simulink model "qdrdac"  (R2012b)
settings: Solver=ode45  StartTime=0.0  StopTime=100  RelTol=1e-3
undefined symbols (not defined in the file or in its folder): pfb_coeff_gen_calc, sfp
undefined symbols (not defined in the file): SL, transtable
libraries: xbsIndex_r4 x4366, casper_library_misc x73, xps_library x14, casper_library_delays x12, maddogLibrary x4, simulink x2
(part 4 of 45)

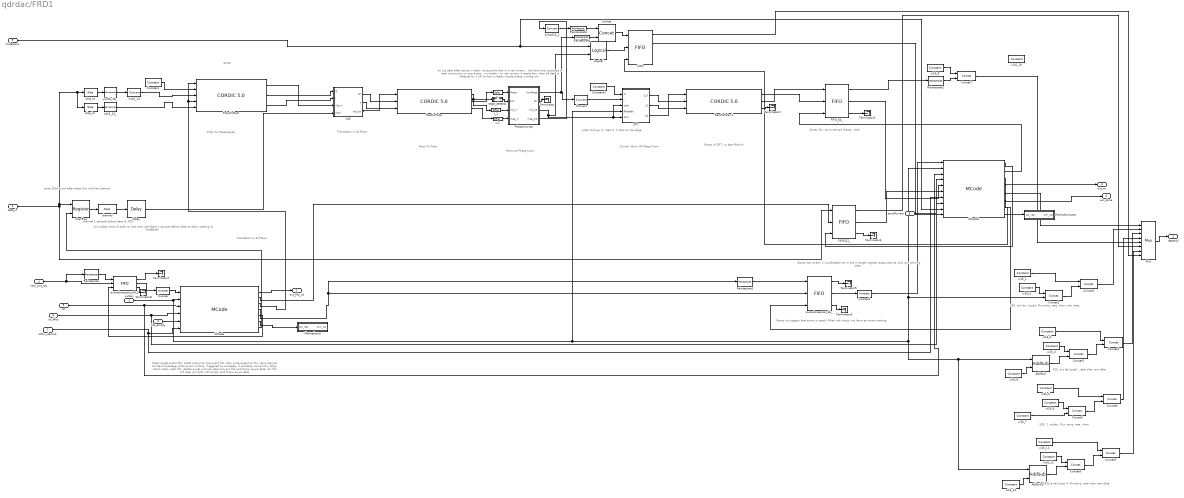
== system qdrdac/FRD1 ==
  note: stroe 32bit word after aaaa
      | this wird has channel
  note: 20 is delay time of polar to rect
      | chan get there 1 sample before data
      | to allow reading of theBRAM
  note: channel 1 sample before
      | data to FRD
  note: Z=20
  note: on 1st data after pause in data, we assume that is a new event...
      | the fsms are supposed to read continuous on one event...no breaks.
      | on new event, it resets fsm. then all data is delayed bu 1 clk so fsm
      | is ready insode phase unwrap ckt.
  note: 555, evt len type1 , aaa chan raw data
  note: 555, evt len, type3, fluxramp, aaa, chan, raw data
  note: 555, 2, evtlen, flux ramp, aaa, chan,
  note: Stores flux ramp dempd [hases. chan
  note: when dvld go hi, start it. it resp to rise edge
  note: Polar To Rectangular
  note: Translation in IQ Plane
  note: Remove Phase Jump
  note: Fourier Xform
      | Of Phase Term
  note: Rect To Polar
  note: Phase of DFT,
      | or Atan(Re/Im)
  note: Translation in IQ Plane
  note: Stores raw event.
      | 2 wordheader
      | len is the in length register
      | aaaa,chan,ts, and raw ph/mag data
  note: Stores up triggers that event is ready
      | When not mptuy we have en event waiting
  note: Read single event fifo.
      | Write output to 2nd event fifo.
      | Also write output to flux ramp demod ckt
      | Send message when event is done.
      | Triggered by evtready. if evtready come from fofop, clrevt ready read fifo.
      | delete evnet will just read sing evt fifo and throw awya data.
      | ckr fifo will clear evt fuifo intil empty and throw awya data
  note: 5555,evlen,type 4, fluxramp, aaa chan tran data
  evtlen : Inport
  fifo_empty : Inport  Port=2
  data_in : Inport  Port=3
  new_evt_rdy : Inport  Port=4
  rst : Inport  Port=5
  clr_fifos : Inport  Port=6
  isflux_demod : Inport  Port=7
  savefluxraw : Inport  Port=8
  circletrans : Inport  Port=9
  AddSub : xbsIndex_r4/AddSub  mode=Addition  use_carryin=off  use_carryout=off  en=off  latency=1  precision=User Defined  arith_type=Unsigned  n_bits=8  bin_pt=0  quantization=Truncate  overflow=Wrap  dbl_ovrd=off  use_behavioral_HDL=off  hw_selection=Fabric  pipelined=off  block_type=addsub
  AddSub1 : xbsIndex_r4/AddSub  mode=Addition  use_carryin=off  use_carryout=off  en=off  latency=1  precision=User Defined  arith_type=Unsigned  n_bits=8  bin_pt=0  quantization=Truncate  overflow=Wrap  dbl_ovrd=off  use_behavioral_HDL=off  hw_selection=Fabric  pipelined=off  block_type=addsub
  Concat{,1..9} (10 alike) : xbsIndex_r4/Concat  num_inputs=2  dbl_ovrd=off  block_type=concat
  Constant : xbsIndex_r4/Constant  const=0  gui_display_data_type=Fixed-point  arith_type=Signed (2's comp)  n_bits=16  bin_pt=14  preci_type=Single  exp_width=8  frac_width=24  explicit_period=on  period=1  equ=P=C  opselect=C  inp2=PCIN>>17  opr=+  inp1=P  carry=CIN  dbl_ovrd=off  block_type=constant
  Constant3 : xbsIndex_r4/Constant  const=0  gui_display_data_type=Fixed-point  arith_type=Signed (2's comp)  n_bits=16  bin_pt=14  preci_type=Single  exp_width=8  frac_width=24  explicit_period=on  period=1  equ=P=C  opselect=C  inp2=PCIN>>17  opr=+  inp1=P  carry=CIN  dbl_ovrd=off  block_type=constant
  Convert : xbsIndex_r4/Convert  gui_display_data_type=Fixed-point  arith_type="Signed  (2's comp)"  n_bits=16  bin_pt=14  float_type=Single  exp_bits=8  fraction_bits=24  quantization=Truncate  overflow=Wrap  en=off  latency=0  dbl_ovrd=off  pipeline=off  block_type=convert
  DFT : Subsystem
  Delay : xbsIndex_r4/Delay  rst=off  infoeditControl=Selection of Reset will increase slice count due to use of real FFs and instead of SRLs  en=off  latency=19  dbl_ovrd=off  reg_retiming=off  block_type=delay
  FIFO : xbsIndex_r4/FIFO  mem_type=Block RAM  performance_options=First_Word_Fall_Through  infoedit1=Available only for V4, V5, V6, V7, K7, A7 and Zynq devices.  embedded_registers=off  depth=512  percent_nbits=1  rst=off  en=off  use_dcount=off  use_percent_full_port=on  use_almost_empty=off  almost_empty_thresh=2  use_almost_full=off  almost_full_thresh=14  dbl_ovrd=off  explicit_period=off  block_type=fifo
  FIFO512_ : xbsIndex_r4/FIFO  mem_type=Block RAM  performance_options=First_Word_Fall_Through  infoedit1=Available only for V4, V5, V6, V7, K7, A7 and Zynq devices.  embedded_registers=off  depth=512  percent_nbits=1  rst=off  en=off  use_dcount=off  use_percent_full_port=off  use_almost_empty=off  almost_empty_thresh=2  use_almost_full=off  almost_full_thresh=256  dbl_ovrd=off  explicit_period=off  block_type=fifo
  FIFO_64_ : xbsIndex_r4/FIFO  mem_type=Block RAM  performance_options=First_Word_Fall_Through  infoedit1=Available only for V4, V5, V6, V7, K7, A7 and Zynq devices.  embedded_registers=off  depth=64  percent_nbits=1  rst=off  en=off  use_dcount=off  use_percent_full_port=off  use_almost_empty=off  almost_empty_thresh=2  use_almost_full=off  almost_full_thresh=32  dbl_ovrd=off  explicit_period=off  block_type=fifo
  Inverter : xbsIndex_r4/Inverter  en=off  latency=0  dbl_ovrd=off  block_type=inv
  Inverter1 : xbsIndex_r4/Inverter  en=off  latency=0  dbl_ovrd=off  block_type=inv
  Logical : xbsIndex_r4/Logical  logical_function=AND  inputs=2  en=off  latency=0  precision=Full  arith_type=Unsigned  n_bits=16  bin_pt=0  align_bp=on  dbl_ovrd=off  block_type=logical
  MCode : xbsIndex_r4/MCode  mfname=fluxRampFSM.m  explicit_period=off  period=1  inputsTable={'boundInpExpr'=>['','','','','',''],'inputs'=>['event_rdy','event_length','rst','clr_fifos','fifo_empty','is_fluxrampdemod']}  outputsTable={'outputs'=>['eventfifo_rd','outfifo_wr','demod_wr','event_done','clr_evt_rdy','stout'],'suppressOut'=>['off','off','off','off','off','off']}  dbl_ovrd=off  enable_stdout=off  enable_debug=off  suppress_output=on  defparams={}  hide_port_list={}  block_type=mcode
  MCode1 : xbsIndex_r4/MCode  mfname=fluxRampFSMOut2  explicit_period=on  period=1  inputsTable={'boundInpExpr'=>['','','','','','','',''],'inputs'=>['event_rdy','event_length','rst','clr_fifos','rawevt_fifo_empty','fluxrmp_fifo_empy','is_fluxrampdemod','is_savefluxraw']}  outputsTable={'outputs'=>['eventfifo_rd','fluxfifo_rd','outfifo_wr','wr_select','event_done','clr_evt_rdy','stout'],'suppressOut'=>['off','off','off','off','off','off','off']}  dbl_ovrd=off  enable_stdout=off  enable_debug=off  suppress_output=on  defparams={}  hide_port_list={}  block_type=mcode
  Mux : xbsIndex_r4/Mux  inputs=7  en=off  latency=0  precision=Full  arith_type=Unsigned  n_bits=16  bin_pt=14  quantization=Truncate  overflow=Wrap  dbl_ovrd=off  block_type=mux
  PhaseUnwrap : Subsystem
  "PolarToRect " : xbsIndex_r4/CORDIC 5.0   functional_selection=Rotate  architectural_configuration=Parallel  pipelining_mode=Maximum  data_format=SignedFraction  phase_format=Scaled_Radians  input_width=16  output_width=16  round_mode=Truncate  iterations=0  precision=0  compensation_scaling=Embedded_Multiplier  coarse_rotation=on  aclken=off  aresetn=off  out_tready=off  cartesian_has_tuser=off  cartesian_has_tlast=off  cartesian_tuser_width=1  phase_has_tuser=off  phase_has_tlast=off  phase_tuser_width=1  out_tlast_behv=Null  flow_control=NonBlocking  optimize_goal=Performance  trim_axipin_name=on  ip_name=CORDIC  ip_version=5.0  dsptool_ready=true  ipcore_usecache=true  ipcore_useipmodelcache=true  wrapper_available=true  port_translation_map={ 'aclken' => 'en', 'aresetn' => 'rst' }  block_type=cordic_v5_0
      settings: infoedit=CORDIC 5.0
  "RectToPolar " : xbsIndex_r4/CORDIC 5.0   functional_selection=Translate  architectural_configuration=Parallel  pipelining_mode=Maximum  data_format=SignedFraction  phase_format=Scaled_Radians  input_width=16  output_width=16  round_mode=Truncate  iterations=0  precision=0  compensation_scaling=Embedded_Multiplier  coarse_rotation=on  aclken=off  aresetn=off  out_tready=off  cartesian_has_tuser=off  cartesian_has_tlast=off  cartesian_tuser_width=1  phase_has_tuser=off  phase_has_tlast=off  phase_tuser_width=1  out_tlast_behv=Null  flow_control=NonBlocking  optimize_goal=Performance  trim_axipin_name=on  ip_name=CORDIC  ip_version=5.0  dsptool_ready=true  ipcore_usecache=true  ipcore_useipmodelcache=true  wrapper_available=true  port_translation_map={ 'aclken' => 'en', 'aresetn' => 'rst' }  block_type=cordic_v5_0
      settings: infoedit=CORDIC 5.0
  RectToPolar 1 : xbsIndex_r4/CORDIC 5.0   functional_selection=Translate  architectural_configuration=Parallel  pipelining_mode=Maximum  data_format=SignedFraction  phase_format=Scaled_Radians  input_width=16  output_width=16  round_mode=Truncate  iterations=0  precision=0  compensation_scaling=Embedded_Multiplier  coarse_rotation=on  aclken=off  aresetn=off  out_tready=off  cartesian_has_tuser=off  cartesian_has_tlast=off  cartesian_tuser_width=1  phase_has_tuser=off  phase_has_tlast=off  phase_tuser_width=1  out_tlast_behv=Null  flow_control=NonBlocking  optimize_goal=Performance  trim_axipin_name=on  ip_name=CORDIC  ip_version=5.0  dsptool_ready=true  ipcore_usecache=true  ipcore_useipmodelcache=true  wrapper_available=true  port_translation_map={ 'aclken' => 'en', 'aresetn' => 'rst' }  block_type=cordic_v5_0
      settings: infoedit=CORDIC 5.0
  Reinterpret : xbsIndex_r4/Reinterpret  force_arith_type=on  arith_type=Unsigned  force_bin_pt=off  bin_pt=0  block_type=reinterpret
  Reinterpret1 : xbsIndex_r4/Reinterpret  force_arith_type=on  arith_type=Unsigned  force_bin_pt=off  bin_pt=0  block_type=reinterpret
  Reinterpret2 : xbsIndex_r4/Reinterpret  force_arith_type=on  arith_type=Unsigned  force_bin_pt=on  bin_pt=0  block_type=reinterpret
  Reinterpret3 : xbsIndex_r4/Reinterpret  force_arith_type=on  arith_type=Unsigned  force_bin_pt=on  bin_pt=0  block_type=reinterpret
  Reinterpret4 : xbsIndex_r4/Reinterpret  force_arith_type=on  arith_type=Unsigned  force_bin_pt=on  bin_pt=0  block_type=reinterpret
  Terminator{,2..8} (8 alike) : Terminator
  chanReg : xbsIndex_r4/Register  init=0  rst=off  en=on  dbl_ovrd=off  block_type=register
  channel : xbsIndex_r4/Slice  nbits=8  boolean_output=off  mode=Lower Bit Location + Width  bit1=0  base1=MSB of Input  bit0=0  base0=LSB of Input  dbl_ovrd=off  block_type=slice
  edge_detect1 : Subsystem  AncestorBlock=casper_library_misc/edge_detect  mask(edge_detect){edge=Rising, polarity=Active High, x_in=[0 0.08 0.08 0.16 0.16 0.24 0.24 0.32 0.32 0.4], y_in=[-1 -1  1  1  1  1  1  1  1  1], x_out=[0.6 0.68 0.68 0.76 0.76 0.84 0.84 0.92 0.92 1], y_out=[-1 -1  1  1 -1 -1 -1 -1 -1 -1]}
      mask prompts: edge "Edge Type"; polarity "Output Polarity"; x_in "Input X Positions"; y_in "Input Y Positions"; x_out "Output X Positions"; y_out "Output Y Positions"
      mask help: Output is active for one-cycle after each edge of the specified type (i.e. rising, falling or both).
      mask init: same as qdrdac/FRD/edge_detect1
      settings: AttributesFormatString=|
      | rising edges
      | active high
      mask Help: Output is active for one-cycle after each edge of the specified type (i.e. rising, falling, or both).  Latency is zero.
      mask TypeOptions edge: Rising | Falling | Both
      mask TypeOptions polarity: Active High | Active Low
      mask Display:
      | plot(x_in_num,0.5+y_in_num*0.2);
      | plot(x_out_num,0.5+y_out_num*0.2);
  evendonequtut_64_ : xbsIndex_r4/FIFO  mem_type=Block RAM  performance_options=First_Word_Fall_Through  infoedit1=Available only for V4, V5, V6, V7, K7, A7 and Zynq devices.  embedded_registers=off  depth=16  percent_nbits=1  rst=off  en=off  use_dcount=off  use_percent_full_port=off  use_almost_empty=off  almost_empty_thresh=2  use_almost_full=off  almost_full_thresh=14  dbl_ovrd=off  explicit_period=off  block_type=fifo
  evendonequtut_64_1 : xbsIndex_r4/FIFO  mem_type=Block RAM  performance_options=First_Word_Fall_Through  infoedit1=Available only for V4, V5, V6, V7, K7, A7 and Zynq devices.  embedded_registers=off  depth=16  percent_nbits=1  rst=off  en=off  use_dcount=off  use_percent_full_port=off  use_almost_empty=off  almost_empty_thresh=2  use_almost_full=off  almost_full_thresh=14  dbl_ovrd=off  explicit_period=off  block_type=fifo
  flrampfsmoutst : Subsystem  Tag=xps:sw_reg  AncestorBlock=xps_library/software register  mask(swreg){mode=one value, io_dir=To Processor, io_delay=0, sample_period=1, names=reg, bitwidths=5, arith_types=0, bin_pts=0, sim_port=on, show_format=off}
      mask prompts: io_dir "I/O direction"; io_delay "I/O delay"; sample_period "Sample period"; names "Name:"; bitwidths "Bitwidth:"; arith_types "Type (ufix=0, fix=1, bool=2):"; bin_pts "Binary pt:"; sim_port "Provide sim input/output?"; show_format "Print format string?"
      mask init:
      | swreg_init(gcb)
      settings: AttributesFormatString=1output
      mask TypeOptions mode: one value | fields of equal size | fields of arbitrary size
      mask Callback mode: swreg_cb(gcb);
      mask TypeOptions io_dir: To Processor | From Processor
      mask Callback io_dir:
      | mask_enables = get_param(gcb, 'MaskEnables');
      | mask_names = get_param(gcb, 'MaskNames');
      | if strcmp(get_param(gcb, 'io_dir'), 'To Processor'),
      |     mask_enables{ismember(mask_names, 'sample_period')} = 'off';
      | else
      |     mask_enables{ismember(mask_names, 'sample_period')} = 'on';
      | end
      | set_param(gcb, 'MaskEnables', mask_enables);
      mask Callback bitwidths:
      | swreg_maskcheck(gcb);
      | % blk = gcb;
      | % mode = get_param(blk, 'mode');
      | % current_widths = eval(get_param(blk, 'bitwidths'));
      | % if (strcmp(mode, 'one value') || strcmp(mode, 'fields of equal size')) && (length(current_widths) > 1),
      | %     error('Only one width may be specified for this mode.');
      | % elseif strcmp(mode, 'fields of arbitrary size')
      | %     current_names = textscan(strtrim(strrep(strrep(get_param(blk, 'names'), ']', ''), '[', '')), '%s');
      | %     current_names = current_names{1};
      | %     numios = length(current_names);
      | %     if length(current_widths) ~= numios,
      | %         error('%d field names specified, but %d widths?', numios, length(current_widths));
      | %     end
      | % end
      | % total_width = 0;
      | % for ctr = 1 : length(current_widths),
      | %     total_width = total_width + current_widths(ctr);
      | % end
      | % if total_width > 32,
      | %     error('Total width must be 32 or less, set to %d.', total_width);
      | % end
      mask Callback arith_types:
      | [numios, ~, ~, ~, current_types] = swreg_maskcheck(gcb);
      | % blk = gcb;
      | % mode = get_param(blk, 'mode');
      | % current_types = eval(get_param(blk, 'arith_types'));
      | % numios = length(current_types);
      | % if (strcmp(mode, 'one value') || strcmp(mode, 'fields of equal size')) && (length(current_types) > 1),
      | %     error('Only one type may be specified for this mode.');
      | % elseif strcmp(mode, 'fields of arbitrary size')
      | %     current_names = textscan(strtrim(strrep(strrep(get_param(blk, 'names'), ']', ''), '[', '')), '%s');
      | %     current_names = current_names{1};
      | %     numios = length(current_names);
      | %     if length(current_types) ~= numios,
      | %         error('%d field names specified, but %d types?', numios, length(current_types));
      | %     end
      | % end
      | problem = 0;
      | for ctr = 1 : numios,
      |     t = current_types(ctr);
      |     if (t < 0) || (t > 2),
      |         problem = t;
      |         ctr = numios + 1;
      |     end
      | end
      | if problem ~= 0,
      |     error('Type cannot be %i, must be 0, 1 or 2.', problem);
      | end
      mask Callback bin_pts:
      | swreg_maskcheck(gcb);
      | % blk = gcb;
      | % mode = get_param(blk, 'mode');
      | % current_bins = eval(get_param(blk, 'bin_pts'));
      | % if (strcmp(mode, 'one value') || strcmp(mode, 'fields of equal size')) && (length(current_bins) > 1),
      | %     error('Only one binary pt may be specified for this mode.');
      | % elseif strcmp(mode, 'fields of arbitrary size')
      | %     current_names = textscan(strtrim(strrep(strrep(get_param(blk, 'names'), ']', ''), '[', '')), '%s');
      | %     current_names = current_names{1};
      | %     numios = length(current_names);
      | %     if length(current_bins) ~= numios,
      | %         error('%d field names specified, but %d binary pts?', numios, length(current_bins));
      | %     end
      | % end
  flrampfsmst : Subsystem  Tag=xps:sw_reg  AncestorBlock=xps_library/software register  mask(swreg){mode=one value, io_dir=To Processor, io_delay=0, sample_period=1, names=reg, bitwidths=4, arith_types=0, bin_pts=0, sim_port=on, show_format=off}
      mask prompts: io_dir "I/O direction"; io_delay "I/O delay"; sample_period "Sample period"; names "Name:"; bitwidths "Bitwidth:"; arith_types "Type (ufix=0, fix=1, bool=2):"; bin_pts "Binary pt:"; sim_port "Provide sim input/output?"; show_format "Print format string?"
      mask init:
      | swreg_init(gcb)
      settings: AttributesFormatString=1output
      mask TypeOptions mode: one value | fields of equal size | fields of arbitrary size
      mask Callback mode: swreg_cb(gcb);
      mask TypeOptions io_dir: To Processor | From Processor
      mask Callback io_dir:
      | mask_enables = get_param(gcb, 'MaskEnables');
      | mask_names = get_param(gcb, 'MaskNames');
      | if strcmp(get_param(gcb, 'io_dir'), 'To Processor'),
      |     mask_enables{ismember(mask_names, 'sample_period')} = 'off';
      | else
      |     mask_enables{ismember(mask_names, 'sample_period')} = 'on';
      | end
      | set_param(gcb, 'MaskEnables', mask_enables);
      mask Callback bitwidths:
      | swreg_maskcheck(gcb);
      | % blk = gcb;
      | % mode = get_param(blk, 'mode');
      | % current_widths = eval(get_param(blk, 'bitwidths'));
      | % if (strcmp(mode, 'one value') || strcmp(mode, 'fields of equal size')) && (length(current_widths) > 1),
      | %     error('Only one width may be specified for this mode.');
      | % elseif strcmp(mode, 'fields of arbitrary size')
      | %     current_names = textscan(strtrim(strrep(strrep(get_param(blk, 'names'), ']', ''), '[', '')), '%s');
      | %     current_names = current_names{1};
      | %     numios = length(current_names);
      | %     if length(current_widths) ~= numios,
      | %         error('%d field names specified, but %d widths?', numios, length(current_widths));
      | %     end
      | % end
      | % total_width = 0;
      | % for ctr = 1 : length(current_widths),
      | %     total_width = total_width + current_widths(ctr);
      | % end
      | % if total_width > 32,
      | %     error('Total width must be 32 or less, set to %d.', total_width);
      | % end
      mask Callback arith_types:
      | [numios, ~, ~, ~, current_types] = swreg_maskcheck(gcb);
      | % blk = gcb;
      | % mode = get_param(blk, 'mode');
      | % current_types = eval(get_param(blk, 'arith_types'));
      | % numios = length(current_types);
      | % if (strcmp(mode, 'one value') || strcmp(mode, 'fields of equal size')) && (length(current_types) > 1),
      | %     error('Only one type may be specified for this mode.');
      | % elseif strcmp(mode, 'fields of arbitrary size')
      | %     current_names = textscan(strtrim(strrep(strrep(get_param(blk, 'names'), ']', ''), '[', '')), '%s');
      | %     current_names = current_names{1};
      | %     numios = length(current_names);
      | %     if length(current_types) ~= numios,
      | %         error('%d field names specified, but %d types?', numios, length(current_types));
      | %     end
      | % end
      | problem = 0;
      | for ctr = 1 : numios,
      |     t = current_types(ctr);
      |     if (t < 0) || (t > 2),
      |         problem = t;
      |         ctr = numios + 1;
      |     end
      | end
      | if problem ~= 0,
      |     error('Type cannot be %i, must be 0, 1 or 2.', problem);
      | end
      mask Callback bin_pts:
      | swreg_maskcheck(gcb);
      | % blk = gcb;
      | % mode = get_param(blk, 'mode');
      | % current_bins = eval(get_param(blk, 'bin_pts'));
      | % if (strcmp(mode, 'one value') || strcmp(mode, 'fields of equal size')) && (length(current_bins) > 1),
      | %     error('Only one binary pt may be specified for this mode.');
      | % elseif strcmp(mode, 'fields of arbitrary size')
      | %     current_names = textscan(strtrim(strrep(strrep(get_param(blk, 'names'), ']', ''), '[', '')), '%s');
      | %     current_names = current_names{1};
      | %     numios = length(current_names);
      | %     if length(current_bins) ~= numios,
      | %         error('%d field names specified, but %d binary pts?', numios, length(current_bins));
      | %     end
      | % end
  int16_13_ : xbsIndex_r4/Reinterpret  force_arith_type=on  arith_type="Signed  (2's comp)"  force_bin_pt=on  bin_pt=13  block_type=reinterpret
      settings: block_version=9.1.01
  int16_14 : xbsIndex_r4/Convert  gui_display_data_type=Fixed-point  arith_type="Signed  (2's comp)"  n_bits=16  bin_pt=14  float_type=Single  exp_bits=8  fraction_bits=24  quantization=Truncate  overflow=Wrap  en=off  latency=0  dbl_ovrd=off  pipeline=off  block_type=convert
  slice_im : xbsIndex_r4/Slice  nbits=16  boolean_output=off  mode=Lower Bit Location + Width  bit1=0  base1=MSB of Input  bit0=0  base0=LSB of Input  dbl_ovrd=off  block_type=slice
      settings: block_version=9.1.01
  slice_re : xbsIndex_r4/Slice  nbits=16  boolean_output=off  mode=Upper Bit Location + Width  bit1=0  base1=MSB of Input  bit0=0  base0=LSB of Input  dbl_ovrd=off  block_type=slice
      settings: block_version=9.1.01
  trIQ : Subsystem
  ui16_{1..2,5,10..11} (5 alike) : xbsIndex_r4/Constant  const=21845  gui_display_data_type=Fixed-point  arith_type=Unsigned  n_bits=16  bin_pt=0  preci_type=Single  exp_width=8  frac_width=24  explicit_period=on  period=1  equ=P=C  opselect=C  inp2=PCIN>>17  opr=+  inp1=P  carry=CIN  dbl_ovrd=off  block_type=constant
  ui16_12 : xbsIndex_r4/Constant  const=4  gui_display_data_type=Fixed-point  arith_type=Unsigned  n_bits=8  bin_pt=0  preci_type=Single  exp_width=8  frac_width=24  explicit_period=on  period=1  equ=P=C  opselect=C  inp2=PCIN>>17  opr=+  inp1=P  carry=CIN  dbl_ovrd=off  block_type=constant
  ui16_13 : xbsIndex_r4/Constant  const=2  gui_display_data_type=Fixed-point  arith_type=Unsigned  n_bits=8  bin_pt=0  preci_type=Single  exp_width=8  frac_width=24  explicit_period=on  period=1  equ=P=C  opselect=C  inp2=PCIN>>17  opr=+  inp1=P  carry=CIN  dbl_ovrd=off  block_type=constant
  ui16_3 : xbsIndex_r4/Constant  const=3  gui_display_data_type=Fixed-point  arith_type=Unsigned  n_bits=8  bin_pt=0  preci_type=Single  exp_width=8  frac_width=24  explicit_period=on  period=1  equ=P=C  opselect=C  inp2=PCIN>>17  opr=+  inp1=P  carry=CIN  dbl_ovrd=off  block_type=constant
  ui16_4 : xbsIndex_r4/Constant  const=1  gui_display_data_type=Fixed-point  arith_type=Unsigned  n_bits=8  bin_pt=0  preci_type=Single  exp_width=8  frac_width=24  explicit_period=on  period=1  equ=P=C  opselect=C  inp2=PCIN>>17  opr=+  inp1=P  carry=CIN  dbl_ovrd=off  block_type=constant
  ui16_6 : xbsIndex_r4/Constant  const=2  gui_display_data_type=Fixed-point  arith_type=Unsigned  n_bits=8  bin_pt=0  preci_type=Single  exp_width=8  frac_width=24  explicit_period=on  period=1  equ=P=C  opselect=C  inp2=PCIN>>17  opr=+  inp1=P  carry=CIN  dbl_ovrd=off  block_type=constant
  ui16_7 : xbsIndex_r4/Constant  const=3  gui_display_data_type=Fixed-point  arith_type=Unsigned  n_bits=8  bin_pt=0  preci_type=Single  exp_width=8  frac_width=24  explicit_period=on  period=1  equ=P=C  opselect=C  inp2=PCIN>>17  opr=+  inp1=P  carry=CIN  dbl_ovrd=off  block_type=constant
  ui16_8 : xbsIndex_r4/Constant  const=2  gui_display_data_type=Fixed-point  arith_type=Unsigned  n_bits=8  bin_pt=0  preci_type=Single  exp_width=8  frac_width=24  explicit_period=on  period=1  equ=P=C  opselect=C  inp2=PCIN>>17  opr=+  inp1=P  carry=CIN  dbl_ovrd=off  block_type=constant
  ui16_9 : xbsIndex_r4/Constant  const=0  gui_display_data_type=Fixed-point  arith_type=Unsigned  n_bits=16  bin_pt=0  preci_type=Single  exp_width=8  frac_width=24  explicit_period=on  period=1  equ=P=C  opselect=C  inp2=PCIN>>17  opr=+  inp1=P  carry=CIN  dbl_ovrd=off  block_type=constant
  uint1616_1 : xbsIndex_r4/Convert  gui_display_data_type=Fixed-point  arith_type=Unsigned  n_bits=16  bin_pt=16  float_type=Single  exp_bits=8  fraction_bits=24  quantization=Truncate  overflow=Wrap  en=off  latency=0  dbl_ovrd=off  pipeline=off  block_type=convert
  uint16_16_ : xbsIndex_r4/Reinterpret  force_arith_type=on  arith_type=Unsigned  force_bin_pt=on  bin_pt=16  block_type=reinterpret
      settings: block_version=9.1.01
  z_ : xbsIndex_r4/Delay  rst=off  infoeditControl=Selection of Reset will increase slice count due to use of real FFs and instead of SRLs  en=off  latency=1  dbl_ovrd=off  reg_retiming=off  block_type=delay
  z_1 : xbsIndex_r4/Delay  rst=off  infoeditControl=Selection of Reset will increase slice count due to use of real FFs and instead of SRLs  en=off  latency=1  dbl_ovrd=off  reg_retiming=off  block_type=delay
  z_2 : xbsIndex_r4/Delay  rst=off  infoeditControl=Selection of Reset will increase slice count due to use of real FFs and instead of SRLs  en=off  latency=1  dbl_ovrd=off  reg_retiming=off  block_type=delay
  evt_fifo_rd : Outport
  dataout : Outport  Port=2
  out_wr : Outport  Port=3
  evt_done : Outport  Port=4
  wires:
  fifo_empty/1 -> MCode/5
  MCode/1 -> evt_fifo_rd/1
  edge_detect1/1(out) -> PhaseUnwrap/2(Rst)
  MCode/4 -> Reinterpret1/1, evendonequtut_64_/2
  "PolarToRect "/1 -> trIQ/3(vld_in)
  DFT/1(Q_F) -> RectToPolar 1/2
  MCode1/4 -> Mux/1
  uint16_16_/1 -> int16_14/1
  FIFO512_/3 -> Terminator4/1
  evendonequtut_64_/3 -> Terminator6/1
  trIQ/3(vld_out) -> "RectToPolar "/1
  evendonequtut_64_/1 -> Terminator5/1
  "RectToPolar "/1 -> z_1/1, edge_detect1/1(in)
  "PolarToRect "/2 -> trIQ/1(Q)
  MCode/5 -> evendonequtut_64_1/3
  "PolarToRect "/3 -> trIQ/2(I)
  "RectToPolar "/3 -> z_2/1
  trIQ/2(It) -> "RectToPolar "/3
  data_in/1 -> slice_im/1, slice_re/1, chanReg/1, FIFO512_/1
  DFT/3(vld) -> RectToPolar 1/1
  Constant/1 -> "PolarToRect "/2
  Constant3/1 -> DFT/1(Q)
  PhaseUnwrap/1(UwrPhase) -> Reinterpret4/1, Convert/1
  PhaseUnwrap/2(Err) -> Terminator/1
  FIFO_64_/2 -> MCode1/6
  rst/1 -> MCode1/3, MCode/3
  evendonequtut_64_1/3 -> Terminator8/1
  MCode1/3 -> out_wr/1
  Inverter1/1 -> MCode1/1
  DFT/2(I_F) -> RectToPolar 1/3
  FIFO512_/2 -> MCode1/5
  MCode1/6 -> evendonequtut_64_/3
  Inverter/1 -> MCode/1
  MCode1/5 -> evt_done/1
  evendonequtut_64_/2 -> Inverter1/1
  evendonequtut_64_1/1 -> Terminator7/1
  RectToPolar 1/3 -> Terminator2/1
  evendonequtut_64_1/2 -> Inverter/1
  PhaseUnwrap/4(mag_out) -> uint1616_1/1
  int16_13_/1 -> "PolarToRect "/5
  clr_fifos/1 -> MCode/4, MCode1/4
  new_evt_rdy/1 -> Reinterpret/1, evendonequtut_64_1/2
  "RectToPolar "/2 -> z_/1
  FIFO_64_/3 -> Terminator3/1
  trIQ/1(Qt) -> "RectToPolar "/2
  MCode1/2 -> FIFO_64_/3
  MCode/2 -> FIFO512_/2
  MCode/3 -> "PolarToRect "/1, "PolarToRect "/4
  isflux_demod/1 -> MCode1/7, MCode/6
  ui16_1/1 -> Concat2/1
  Concat1/1 -> Concat2/2
  ui16_3/1 -> Concat1/1
  Concat2/1 -> Mux/2
  Concat7/1 -> Mux/5
  FIFO512_/1 -> Mux/6
  ui16_2/1 -> Concat4/1
  Concat3/1 -> Concat4/2
  ui16_4/1 -> Concat3/1
  ui16_5/1 -> Concat6/1
  Concat5/1 -> Concat6/2
  ui16_6/1 -> Concat5/1
  ui16_7/1 -> Concat5/2
  Concat4/1 -> Mux/3
  Concat6/1 -> Mux/4
  ui16_8/1 -> AddSub/2
  AddSub/1 -> Concat3/2
  savefluxraw/1 -> MCode1/8
  Reinterpret/1 -> evendonequtut_64_1/1
  Reinterpret1/1 -> evendonequtut_64_/1
  RectToPolar 1/1 -> FIFO_64_/2
  RectToPolar 1/2 -> FIFO_64_/1
  MCode1/1 -> FIFO512_/3
  Mux/1 -> dataout/1
  Reinterpret2/1 -> Concat7/2
  FIFO_64_/1 -> Reinterpret2/1
  ui16_9/1 -> Concat7/1
  slice_re/1 -> uint16_16_/1
  slice_im/1 -> int16_13_/1
  int16_14/1 -> "PolarToRect "/3
  MCode1/7 -> flrampfsmoutst/1(out_reg)
  z_1/1 -> PhaseUnwrap/3(vld_in)
  z_2/1 -> PhaseUnwrap/4(mag_in)
  z_/1 -> PhaseUnwrap/1(Phase)
  MCode/6 -> flrampfsmst/1(out_reg)
  MCode/7 -> chanReg/2
  chanReg/1 -> channel/1
  channel/1 -> Delay/1
  Delay/1 -> trIQ/4(chan)
  Concat/1 -> FIFO/1
  PhaseUnwrap/3(vld_out) -> Logical/2, DFT/3(start), DFT/5(dvld)
  Logical/1 -> FIFO/2
  FIFO/2 -> MCode1/10
  circletrans/1 -> MCode1/9, Logical/1
  ui16_11/1 -> Concat9/1
  Concat8/1 -> Concat9/2
  ui16_12/1 -> Concat8/1
  evtlen/1 -> MCode/2, DFT/4(fftlen8bit), Concat1/2, MCode1/2, AddSub1/1, AddSub/1
  ui16_13/1 -> AddSub1/2
  AddSub1/1 -> Concat8/2
  Concat9/1 -> Mux/7
  FIFO/1 -> Mux/8
  MCode1/8 -> FIFO/3
  Reinterpret4/1 -> Concat/2
  Reinterpret3/1 -> Concat/1
  Convert/1 -> DFT/2(I)
  uint1616_1/1 -> Reinterpret3/1

== system qdrdac/FineMix ==
  In1 : Inport
  In2 : Inport  Port=2
  In3 : Inport  Port=3
  In4 : Inport  Port=4
  In5 : Inport  Port=5
  In6 : Inport  Port=6
  In7 : Inport  Port=7
  In8 : Inport  Port=8
  In9 : Inport  Port=9
  In11 : Inport  Port=10
  In12 : Inport  Port=11
  In13 : Inport  Port=12
  In16 : Inport  Port=13
  PhaseCorrect3 : Subsystem
  PhaseCorrect4 : Subsystem
  PhaseCorrect5 : Subsystem
  PhaseCorrect6 : Subsystem
  rect2polarV1 : Subsystem
  rect2polarV2 : Subsystem
  rect2polarV3 : Subsystem
  rect2polarV5 : Subsystem
  chanout1 : Outport
  dvalout1 : Outport  Port=2
  dout1 : Outport  Port=3
  chanout2 : Outport  Port=4
  dvalout2 : Outport  Port=5
  dout2 : Outport  Port=6
  dvldout3 : Outport  Port=7
  chanout3 : Outport  Port=8
  dvldout4 : Outport  Port=9
  dout3 : Outport  Port=10
  chanout4 : Outport  Port=11
  dout4 : Outport  Port=12
  wires:
  In9/1 -> rect2polarV5/2(cmplx)
  In11/1 -> rect2polarV1/2(cmplx)
  In13/1 -> rect2polarV3/2(cmplx)
  In12/1 -> rect2polarV2/2(cmplx)
  In1/1 -> rect2polarV5/1(dvalid)
  In2/1 -> rect2polarV1/1(dvalid)
  In3/1 -> rect2polarV2/1(dvalid)
  In4/1 -> rect2polarV3/1(dvalid)
  In5/1 -> rect2polarV5/3(chan)
  In6/1 -> rect2polarV1/3(chan)
  In7/1 -> rect2polarV2/3(chan)
  In8/1 -> rect2polarV3/3(chan)
  PhaseCorrect4/3(chanout) -> chanout2/1
  PhaseCorrect3/2(cmplx_dout) -> dout1/1
  PhaseCorrect4/2(cmplx_dout) -> dout2/1
  PhaseCorrect3/3(chanout) -> chanout1/1
  PhaseCorrect5/2(cmplx_dout) -> dout3/1
  PhaseCorrect6/2(cmplx_dout) -> dout4/1
  PhaseCorrect5/3(chanout) -> chanout3/1
  PhaseCorrect6/3(chanout) -> chanout4/1
  PhaseCorrect3/1(dvld_out) -> dvalout1/1
  PhaseCorrect4/1(dvld_out) -> dvalout2/1
  PhaseCorrect5/1(dvld_out) -> dvldout3/1
  PhaseCorrect6/1(dvld_out) -> dvldout4/1
  rect2polarV5/1(dvalidout) -> PhaseCorrect3/1(dvld_in)
  rect2polarV5/2(pol) -> PhaseCorrect3/2(cmplx_din)
  rect2polarV5/3(chandly) -> PhaseCorrect3/3(chan)
  rect2polarV1/1(dvalidout) -> PhaseCorrect4/1(dvld_in)
  rect2polarV1/2(pol) -> PhaseCorrect4/2(cmplx_din)
  rect2polarV1/3(chandly) -> PhaseCorrect4/3(chan)
  rect2polarV2/3(chandly) -> PhaseCorrect5/3(chan)
  rect2polarV2/2(pol) -> PhaseCorrect5/2(cmplx_din)
  rect2polarV2/1(dvalidout) -> PhaseCorrect5/1(dvld_in)
  rect2polarV3/3(chandly) -> PhaseCorrect6/3(chan)
  rect2polarV3/2(pol) -> PhaseCorrect6/2(cmplx_din)
  rect2polarV3/1(dvalidout) -> PhaseCorrect6/1(dvld_in)
  In16/1 -> PhaseCorrect5/4(rstAccum), PhaseCorrect4/4(rstAccum), PhaseCorrect3/4(rstAccum), PhaseCorrect6/4(rstAccum)

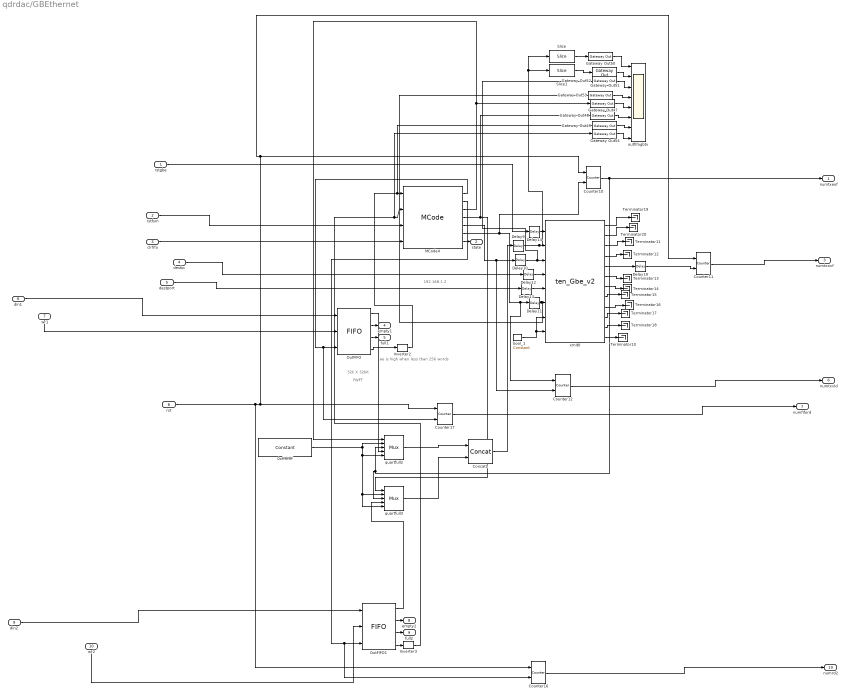
== system qdrdac/GBEthernet ==
  note: ae is high when less than 256 words
  note: FWFT
  note: 32k X 32bit
  note: 192.168.1.2
  rstgbe : Inport
  rstfsm : Inport  Port=2
  clrfifo : Inport  Port=3
  destip : Inport  Port=4
  destport : Inport  Port=5
  din1 : Inport  Port=6
  wr1 : Inport  Port=7
  rst : Inport  Port=8
  din2 : Inport  Port=9
  wr2 : Inport  Port=10
  0xffffffff : xbsIndex_r4/Constant  const=hex2dec('ffffffff')  gui_display_data_type=Fixed-point  arith_type=Unsigned  n_bits=32  bin_pt=0  preci_type=Single  exp_width=8  frac_width=24  explicit_period=on  period=1  equ=P=C  opselect=C  inp2=PCIN>>17  opr=+  inp1=P  carry=CIN  dbl_ovrd=off  block_type=constant
  Concat1 : xbsIndex_r4/Concat  num_inputs=2  dbl_ovrd=off  block_type=concat
  Counter{10..12,16..17} (5 alike) : xbsIndex_r4/Counter  cnt_type=Free Running  cnt_to=Inf  operation=Up  start_count=0  cnt_by_val=1  arith_type=Unsigned  n_bits=32  bin_pt=0  load_pin=off  rst=on  en=on  explicit_period=on  period=1  dbl_ovrd=off  use_behavioral_HDL=off  implementation=Fabric  block_type=counter
  Delay{9..14,19} (7 alike) : xbsIndex_r4/Delay  rst=off  infoeditControl=Selection of Reset will increase slice count due to use of real FFs and instead of SRLs  en=off  latency=1  dbl_ovrd=off  reg_retiming=off  block_type=delay
  Gateway Out{47..54} (8 alike) : xbsIndex_r4/Gateway Out  inherit_from_input=off  hdl_port=on  timing_constraint=None  locs_specified=off  LOCs={}  UseAsDAC=off  DACChannel='1'  block_type=gatewayout
  Inverter2 : xbsIndex_r4/Inverter  en=off  latency=0  dbl_ovrd=off  block_type=inv
  Inverter3 : xbsIndex_r4/Inverter  en=off  latency=0  dbl_ovrd=off  block_type=inv
  MCode4 : xbsIndex_r4/MCode  mfname=gbDataWrite  explicit_period=off  period=1  inputsTable={'boundInpExpr'=>['','',''],'inputs'=>['almost_empty_a','almost_empty_b','rst']}  outputsTable={'outputs'=>['fifo_rd_a','fifo_rd_b','mux_a','mux_b','tx_vld','tx_eof','stateout'],'suppressOut'=>['off','off','off','off','off','off','off']}  dbl_ovrd=off  enable_stdout=off  enable_debug=off  suppress_output=on  defparams={}  hide_port_list={}  block_type=mcode
  OutFIFO : xbsIndex_r4/FIFO  mem_type=Block RAM  performance_options=First_Word_Fall_Through  infoedit1=Available only for V4, V5, V6, V7, K7, A7 and Zynq devices.  embedded_registers=off  depth=32K  percent_nbits=1  rst=off  en=off  use_dcount=off  use_percent_full_port=off  use_almost_empty=on  almost_empty_thresh=256  use_almost_full=off  almost_full_thresh=14  dbl_ovrd=off  explicit_period=off  block_type=fifo
  OutFIFO1 : xbsIndex_r4/FIFO  mem_type=Block RAM  performance_options=First_Word_Fall_Through  infoedit1=Available only for V4, V5, V6, V7, K7, A7 and Zynq devices.  embedded_registers=off  depth=32K  percent_nbits=1  rst=off  en=off  use_dcount=off  use_percent_full_port=off  use_almost_empty=on  almost_empty_thresh=256  use_almost_full=off  almost_full_thresh=14  dbl_ovrd=off  explicit_period=off  block_type=fifo
  Slice : xbsIndex_r4/Slice  nbits=32  boolean_output=off  mode=Lower Bit Location + Width  bit1=0  base1=MSB of Input  bit0=0  base0=LSB of Input  dbl_ovrd=off  block_type=slice
  Slice1 : xbsIndex_r4/Slice  nbits=32  boolean_output=off  mode=Upper Bit Location + Width  bit1=0  base1=MSB of Input  bit0=0  base0=LSB of Input  dbl_ovrd=off  block_type=slice
  Terminator{10..20} (11 alike) : Terminator
  bool_1 : xbsIndex_r4/Constant  const=0  gui_display_data_type=Boolean  arith_type=Boolean  n_bits=16  bin_pt=14  preci_type=Single  exp_width=8  frac_width=24  explicit_period=on  period=1  equ=P=C  opselect=C  inp2=PCIN>>17  opr=+  inp1=P  carry=CIN  dbl_ovrd=off  block_type=constant
  outfifogbtx : Scope  NumInputPorts=8
      settings: YMin=-5~-5~-5~-5~-5~-5~-5~-5  YMax=5~5~5~5~5~5~5~5  SaveName=outfifodata
  quartfull2 : xbsIndex_r4/Mux  inputs=4  en=off  latency=0  precision=Full  arith_type=Unsigned  n_bits=16  bin_pt=14  quantization=Truncate  overflow=Wrap  dbl_ovrd=off  block_type=mux
  quartfull3 : xbsIndex_r4/Mux  inputs=4  en=off  latency=0  precision=Full  arith_type=Unsigned  n_bits=16  bin_pt=14  quantization=Truncate  overflow=Wrap  dbl_ovrd=off  block_type=mux
  xmit0 : xps_library/ten_Gbe_v2  Tag=xps:tengbe_v2  flavour=sfp+  slot=1  port_r1=0  port_r2_cx4=0  port_r2_sfpp=0  rx_dist_ram=off  large_frames=off  show_param=off  pre_emph_r2=1.07  pre_emph=3  post_emph_r2=0.18  rxeqmix_r2=7  swing_r2=940  swing=800  fab_en=on  fab_mac=hex2dec('123456780000')  fab_ip=192*(2^24) + 168*(2^16) + 5*(2^8) + 20*(2^0)  fab_udp=10000  fab_gate=1  cpu_rx_en=on  cpu_tx_en=on  ttl=hex2dec('FF')  promisc_mode=off  debug_ctr_width=16  txctr=off  txerrctr=off  txerrctr_len=100  txofctr=off  txfullctr=off  txvldctr=off  txsnaplen=0 - no snap  rxctr=off  rxerrctr=off  rxerrctr_len=100  rxofctr=off  rxbadctr=off  rxvldctr=off  rxeofctr=off  rxsnaplen=0 - no snap
  numtxeof : Outport
  state : Outport  Port=2
  numtxovf : Outport  Port=3
  empty1 : Outport  Port=4
  full1 : Outport  Port=5
  numtxvld : Outport  Port=6
  numfiford : Outport  Port=7
  empty2 : Outport  Port=8
  full2 : Outport  Port=9
  numrd2 : Outport  Port=10
  wires:
  xmit0/1 -> Terminator19/1
  wr2/1 -> OutFIFO1/2
  xmit0/6 -> Terminator13/1
  wr1/1 -> OutFIFO/2
  OutFIFO1/3 -> full2/1
  xmit0/8 -> Terminator15/1
  xmit0/2 -> Terminator20/1
  xmit0/9 -> Terminator16/1
  xmit0/3 -> Terminator11/1
  OutFIFO/2 -> empty1/1
  OutFIFO/3 -> full1/1
  MCode4/7 -> state/1
  xmit0/10 -> Terminator17/1
  OutFIFO1/2 -> empty2/1
  xmit0/7 -> Terminator14/1
  xmit0/4 -> Terminator12/1
  xmit0/11 -> Terminator18/1
  xmit0/12 -> Terminator10/1
  destip/1 -> Delay12/1
  destport/1 -> Delay13/1
  Concat1/1 -> Delay9/1
  bool_1/1 -> xmit0/8, xmit0/7
  xmit0/5 -> Delay19/1
  MCode4/5 -> Counter12/2, Delay10/1
  Inverter2/1 -> Gateway Out49/1, MCode4/1
  rstfsm/1 -> MCode4/3
  MCode4/2 -> Counter16/2, OutFIFO1/3
  0xffffffff/1 -> quartfull2/5, quartfull3/5, quartfull3/2, quartfull2/2
  OutFIFO1/1 -> quartfull3/4
  OutFIFO1/4 -> Inverter3/1
  OutFIFO/1 -> quartfull2/4
  MCode4/3 -> Gateway Out47/1, quartfull2/1
  MCode4/4 -> Gateway Out48/1, quartfull3/1
  quartfull2/1 -> Concat1/1
  quartfull3/1 -> Concat1/2
  MCode4/1 -> Counter17/2, OutFIFO/3
  Delay9/1 -> Slice1/1, Slice/1, xmit0/2
  Delay10/1 -> Gateway Out52/1, xmit0/3
  Delay11/1 -> Gateway Out53/1, xmit0/6
  Delay12/1 -> xmit0/4
  rstgbe/1 -> Delay14/1
  Delay13/1 -> xmit0/5
  Delay14/1 -> xmit0/1
  Delay19/1 -> Counter11/2
  OutFIFO/4 -> Inverter2/1
  Inverter3/1 -> Gateway Out54/1, MCode4/2
  MCode4/6 -> Counter10/2, Counter12/1, Delay11/1
  Counter11/1 -> numtxovf/1
  Counter12/1 -> numtxvld/1
  rst/1 -> Counter11/1, Counter10/1, Counter17/1, Counter16/1
  Counter10/1 -> numtxeof/1, quartfull2/3, quartfull3/3
  clrfifo/1 -> MCode4/4
  Counter16/1 -> numrd2/1
  Counter17/1 -> numfiford/1
  Gateway Out53/1 -> outfifogbtx/4
  Gateway Out50/1 -> outfifogbtx/1
  Gateway Out48/1 -> outfifogbtx/6
  Gateway Out52/1 -> outfifogbtx/3
  Gateway Out49/1 -> outfifogbtx/7
  Gateway Out54/1 -> outfifogbtx/8
  Gateway Out51/1 -> outfifogbtx/2
  Gateway Out47/1 -> outfifogbtx/5
  Slice/1 -> Gateway Out50/1
  Slice1/1 -> Gateway Out51/1
  din1/1 -> OutFIFO/1
  din2/1 -> OutFIFO1/1

== system qdrdac/MKID_ADC ==
  in128 : Inport
  Constant : Constant
  Mux{,1..7} (8 alike) : xbsIndex_r4/Mux  inputs=2  en=off  latency=1  precision=Full  arith_type=Unsigned  n_bits=16  bin_pt=14  quantization=Truncate  overflow=Wrap  dbl_ovrd=off  block_type=mux
  adc_mkid_4x_r2 : xps_library/ADCs/adc_mkid_4x_r2  Tag=xps:adc_mkid_4x_r2  adc_clk_rate=512
  bit0_ : xbsIndex_r4/Slice  nbits=0  boolean_output=on  mode=Lower Bit Location + Width  bit1=0  base1=MSB of Input  bit0=0  base0=LSB of Input  dbl_ovrd=off  block_type=slice
  buss128toIQ1 : Subsystem
  fix12_11_{1..8} (8 alike) : xbsIndex_r4/Reinterpret  force_arith_type=on  arith_type="Signed  (2's comp)"  force_bin_pt=on  bin_pt=11  block_type=reinterpret
  settings : Subsystem  Tag=xps:sw_reg  AncestorBlock=xps_library/software register  mask(swreg){mode=one value, io_dir=From Processor, io_delay=0, sample_period=1, names=reg, bitwidths=32, arith_types=0, bin_pts=0, sim_port=on, show_format=off}
      mask prompts: io_dir "I/O direction"; io_delay "I/O delay"; sample_period "Sample period"; names "Name:"; bitwidths "Bitwidth:"; arith_types "Type (ufix=0, fix=1, bool=2):"; bin_pts "Binary pt:"; sim_port "Provide sim input/output?"; show_format "Print format string?"
      mask init:
      | swreg_init(gcb)
      settings: AttributesFormatString=1input
      mask TypeOptions mode: one value | fields of equal size | fields of arbitrary size
      mask Callback mode: swreg_cb(gcb);
      mask TypeOptions io_dir: To Processor | From Processor
      mask Callback io_dir:
      | mask_enables = get_param(gcb, 'MaskEnables');
      | mask_names = get_param(gcb, 'MaskNames');
      | if strcmp(get_param(gcb, 'io_dir'), 'To Processor'),
      |     mask_enables{ismember(mask_names, 'sample_period')} = 'off';
      | else
      |     mask_enables{ismember(mask_names, 'sample_period')} = 'on';
      | end
      | set_param(gcb, 'MaskEnables', mask_enables);
      mask Callback bitwidths:
      | swreg_maskcheck(gcb);
      | % blk = gcb;
      | % mode = get_param(blk, 'mode');
      | % current_widths = eval(get_param(blk, 'bitwidths'));
      | % if (strcmp(mode, 'one value') || strcmp(mode, 'fields of equal size')) && (length(current_widths) > 1),
      | %     error('Only one width may be specified for this mode.');
      | % elseif strcmp(mode, 'fields of arbitrary size')
      | %     current_names = textscan(strtrim(strrep(strrep(get_param(blk, 'names'), ']', ''), '[', '')), '%s');
      | %     current_names = current_names{1};
      | %     numios = length(current_names);
      | %     if length(current_widths) ~= numios,
      | %         error('%d field names specified, but %d widths?', numios, length(current_widths));
      | %     end
      | % end
      | % total_width = 0;
      | % for ctr = 1 : length(current_widths),
      | %     total_width = total_width + current_widths(ctr);
      | % end
      | % if total_width > 32,
      | %     error('Total width must be 32 or less, set to %d.', total_width);
      | % end
      mask Callback arith_types:
      | [numios, ~, ~, ~, current_types] = swreg_maskcheck(gcb);
      | % blk = gcb;
      | % mode = get_param(blk, 'mode');
      | % current_types = eval(get_param(blk, 'arith_types'));
      | % numios = length(current_types);
      | % if (strcmp(mode, 'one value') || strcmp(mode, 'fields of equal size')) && (length(current_types) > 1),
      | %     error('Only one type may be specified for this mode.');
      | % elseif strcmp(mode, 'fields of arbitrary size')
      | %     current_names = textscan(strtrim(strrep(strrep(get_param(blk, 'names'), ']', ''), '[', '')), '%s');
      | %     current_names = current_names{1};
      | %     numios = length(current_names);
      | %     if length(current_types) ~= numios,
      | %         error('%d field names specified, but %d types?', numios, length(current_types));
      | %     end
      | % end
      | problem = 0;
      | for ctr = 1 : numios,
      |     t = current_types(ctr);
      |     if (t < 0) || (t > 2),
      |         problem = t;
      |         ctr = numios + 1;
      |     end
      | end
      | if problem ~= 0,
      |     error('Type cannot be %i, must be 0, 1 or 2.', problem);
      | end
      mask Callback bin_pts:
      | swreg_maskcheck(gcb);
      | % blk = gcb;
      | % mode = get_param(blk, 'mode');
      | % current_bins = eval(get_param(blk, 'bin_pts'));
      | % if (strcmp(mode, 'one value') || strcmp(mode, 'fields of equal size')) && (length(current_bins) > 1),
      | %     error('Only one binary pt may be specified for this mode.');
      | % elseif strcmp(mode, 'fields of arbitrary size')
      | %     current_names = textscan(strtrim(strrep(strrep(get_param(blk, 'names'), ']', ''), '[', '')), '%s');
      | %     current_names = current_names{1};
      | %     numios = length(current_names);
      | %     if length(current_bins) ~= numios,
      | %         error('%d field names specified, but %d binary pts?', numios, length(current_bins));
      | %     end
      | % end
  top12_{0..7} (8 alike) : xbsIndex_r4/Slice  nbits=12  boolean_output=off  mode=Upper Bit Location + Width  bit1=0  base1=MSB of Input  bit0=0  base0=LSB of Input  dbl_ovrd=off  block_type=slice
  i0 : Outport
  i1 : Outport  Port=2
  i2 : Outport  Port=3
  i3 : Outport  Port=4
  q0 : Outport  Port=5
  q1 : Outport  Port=6
  q2 : Outport  Port=7
  q3 : Outport  Port=8
  sync : Outport  Port=9
  wires:
  adc_mkid_4x_r2/9 -> sync/1
  buss128toIQ1/1(I0) -> top12_0/1
  buss128toIQ1/2(I1) -> top12_1/1
  buss128toIQ1/3(I2) -> top12_2/1
  buss128toIQ1/4(I3) -> top12_3/1
  buss128toIQ1/5(Q0) -> top12_4/1
  buss128toIQ1/6(Q1) -> top12_5/1
  buss128toIQ1/7(Q2) -> top12_6/1
  buss128toIQ1/8(Q3) -> top12_7/1
  top12_0/1 -> fix12_11_8/1
  top12_1/1 -> fix12_11_7/1
  top12_2/1 -> fix12_11_6/1
  top12_3/1 -> fix12_11_5/1
  top12_4/1 -> fix12_11_4/1
  top12_5/1 -> fix12_11_3/1
  top12_6/1 -> fix12_11_2/1
  top12_7/1 -> fix12_11_1/1
  adc_mkid_4x_r2/1 -> Mux/2
  adc_mkid_4x_r2/2 -> Mux1/2
  adc_mkid_4x_r2/3 -> Mux2/2
  adc_mkid_4x_r2/4 -> Mux3/2
  adc_mkid_4x_r2/5 -> Mux4/2
  adc_mkid_4x_r2/6 -> Mux5/2
  adc_mkid_4x_r2/7 -> Mux6/2
  adc_mkid_4x_r2/8 -> Mux7/2
  in128/1 -> buss128toIQ1/1(In1)
  settings/1(in_reg) -> bit0_/1
  bit0_/1 -> Mux1/1, Mux/1, Mux2/1, Mux3/1, Mux4/1, Mux5/1, Mux6/1, Mux7/1
  Constant/1 -> settings/1(sim_1)
  fix12_11_8/1 -> Mux/3
  fix12_11_7/1 -> Mux1/3
  fix12_11_6/1 -> Mux2/3
  fix12_11_5/1 -> Mux3/3
  fix12_11_4/1 -> Mux4/3
  fix12_11_3/1 -> Mux5/3
  fix12_11_2/1 -> Mux6/3
  fix12_11_1/1 -> Mux7/3
  Mux/1 -> i0/1
  Mux1/1 -> i1/1
  Mux2/1 -> i2/1
  Mux3/1 -> i3/1
  Mux4/1 -> q0/1
  Mux5/1 -> q1/1
  Mux6/1 -> q2/1
  Mux7/1 -> q3/1
